simulink model "KompezacijaNepotpunaTabela"  (R2016b)
settings: Solver=VariableStepAuto  StartTime=0.0  StopTime=800  RelTol=1e-3
libraries: simulink x1
settings Model: Creator=Luka  LastModifiedBy=Luka

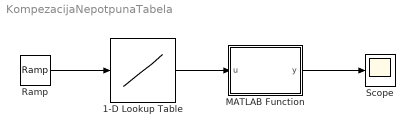
== system KompezacijaNepotpunaTabela ==
  1-D Lookup Table : Lookup_n-D  NumberOfTableDimensions=1  BreakpointsForDimension1=[0 100 200 300 400 500 600 700 800]  Table=[0 19.673 31.606 38.843 43.233 45.896 47.511 48.490 49.084]  InternalRulePriority=Speed  RndMeth=Simplest  InputSameDT=on
  MATLAB Function : MATLAB Function  TreatAsAtomicUnit=on
  Ramp : simulink/Sources/Ramp  slope=1  start=0  X0=0
  Scope : Scope
  wires:
  Ramp/1 -> 1-D Lookup Table/1
  1-D Lookup Table/1 -> MATLAB Function/1(u)
  MATLAB Function/1(y) -> Scope/1

== matlab function KompezacijaNepotpunaTabela/MATLAB Function ==
  data: u input; y output
function y = fcn(u)

y = -200*log(1 - u/50);
